simulink model "train_ras"  (R2023b)
settings: Solver=VariableStepAuto  StartTime=0.0  StopTime=20  MaxStep=0.01  RelTol=1e-3
values from neighbouring files (symbols this model uses):
  a1 = 2    [pid_ras.m]
  a2 = 2    [pid_ras.m]
  b = 0.5    [pid_ras.m]
  c = 0.75    [pid_ras.m]
  Kd = 7    [pid_ras.m]
  Ki = 9    [pid_ras.m]
  Kp = 15    [pid_ras.m]
  xref = 5    [pid_ras.m]
settings Model: Creator=eleft  LastModifiedBy=jimkam

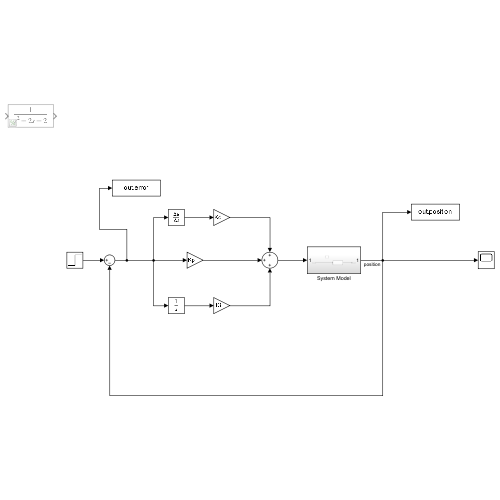
[thumbnail: Simulink's stored preview of the top-level diagram]
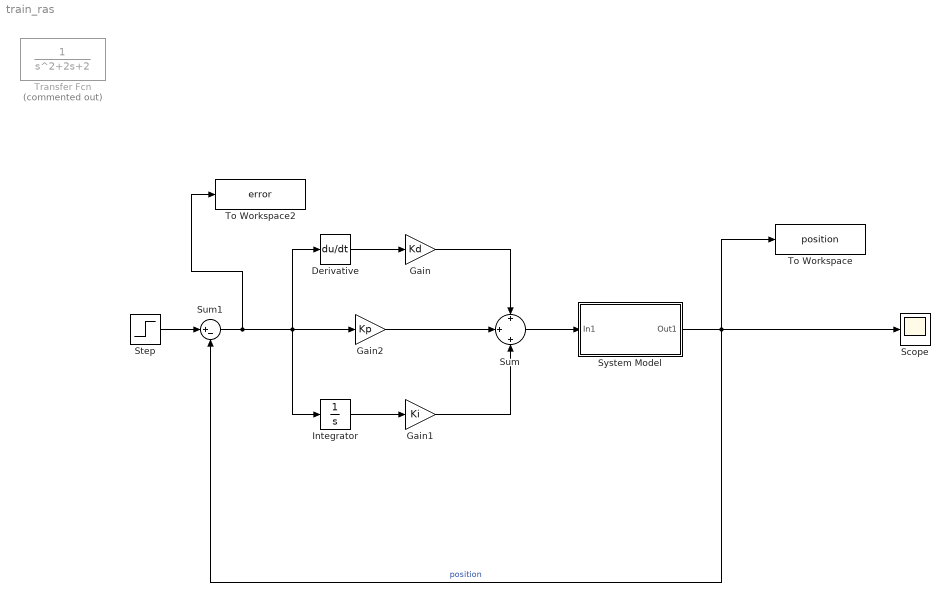
== system train_ras ==
  Derivative : Derivative  CoefficientInTFapproximation=0
  Gain : Gain  Gain=Kd
  Gain1 : Gain  Gain=Ki
  Gain2 : Gain  Gain=Kp
  Integrator : Integrator
  Scope : Scope
  Step : Step  After=xref  SampleTime=0
  Sum : Sum  Inputs=+|+|+
  Sum1 : Sum  Inputs=|+-
  System Model : Subsystem
  To Workspace : ToWorkspace  VariableName=position  SaveFormat=Timeseries  SampleTime=-1
      settings: Decimation=2
  To Workspace2 : ToWorkspace  VariableName=error  SaveFormat=Timeseries  SampleTime=-1
  Transfer Fcn : TransferFcn  Commented=on  Denominator=[1 2 2]
  wires:
  Derivative/1 -> Gain/1
  Gain/1 -> Sum/1
  Gain2/1 -> Sum/2
  Gain1/1 -> Sum/3
  Integrator/1 -> Gain1/1
  Sum1/1 -> To Workspace2/1, Integrator/1, Derivative/1, Gain2/1
  Sum/1 -> System Model/1(In1)
  Step/1 -> Sum1/1
  System Model/1(Out1) -> To Workspace/1, Scope/1, Sum1/2  "position"

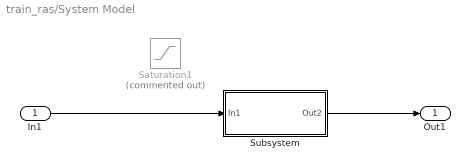
== system train_ras/System Model ==
  In1 : Inport
  Saturation1 : Saturate  Commented=on  UpperLimit=1  LowerLimit=-1
  Subsystem : Subsystem
  Out1 : Outport
  wires:
  In1/1 -> Subsystem/1(In1)
  Subsystem/1(Out2) -> Out1/1

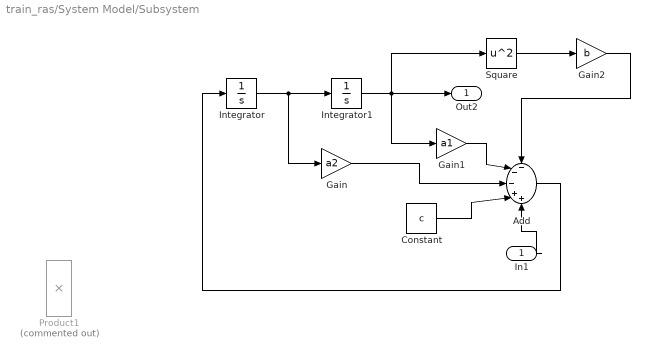
== system train_ras/System Model/Subsystem ==
  In1 : Inport
  Add : Sum  Inputs=---++
  Constant : Constant  Value=c
  Gain : Gain  Gain=a2
  Gain1 : Gain  Gain=a1
  Gain2 : Gain  Gain=b
  Integrator : Integrator
  Integrator1 : Integrator
  Product1 : Product  Commented=on
  Square : Math  Operator=square
  Out2 : Outport
  wires:
  Integrator1/1 -> Square/1, Out2/1, Gain1/1
  Integrator/1 -> Gain/1, Integrator1/1
  Add/1 -> Integrator/1
  In1/1 -> Add/5
  Gain/1 -> Add/3
  Gain1/1 -> Add/2
  Square/1 -> Gain2/1
  Gain2/1 -> Add/1
  Constant/1 -> Add/4
